simulink model "ControlCorrientePR"  (R2019a)
settings: Solver=VariableStepAuto  StartTime=0.0  StopTime=10.0  RelTol=1e-3
libraries: cstblocks x4
settings Model: Creator=Seba Morales  LastModifiedBy=Seba Morales

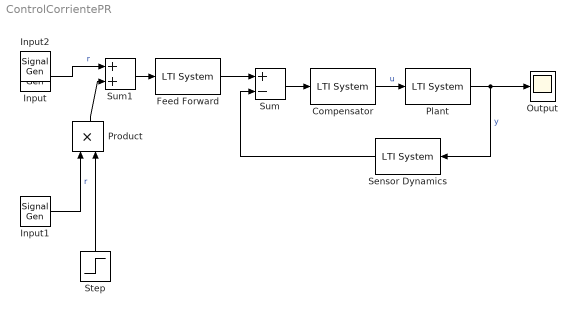
== system ControlCorrientePR ==
  Compensator : cstblocks/LTI System  sys=C  IC=[]
  Feed Forward : cstblocks/LTI System  sys=F  IC=[]
  Input : SignalGenerator  Amplitude=60  Frequency=50
  Input1 : SignalGenerator  Amplitude=30  Frequency=50
  Input2 : SignalGenerator  Amplitude=60  Frequency=50
  Output : Scope
  Plant : cstblocks/LTI System  sys=G  IC=[]
  Product : Product
  Sensor Dynamics : cstblocks/LTI System  sys=H  IC=[]
  Step : Step  SampleTime=0
  Sum : Sum  Inputs=+-  SaturateOnIntegerOverflow=on  InputSameDT=on  OutDataTypeStr=Inherit: Same as first input
  Sum1 : Sum  SaturateOnIntegerOverflow=on  InputSameDT=on  OutDataTypeStr=Inherit: Same as first input
  wires:
  Feed Forward/1 -> Sum/1
  Sensor Dynamics/1 -> Sum/2
  Sum/1 -> Compensator/1
  Compensator/1 -> Plant/1  "u"
  Plant/1 -> Output/1, Sensor Dynamics/1  "y"
  Sum1/1 -> Feed Forward/1
  Input/1 -> Sum1/1  "r"
  Product/1 -> Sum1/2
  Step/1 -> Product/2
  Input1/1 -> Product/1  "r"
